simulink model "NonLinearFunction"  (R2021a)
settings: Solver=VariableStepAuto  StartTime=0.0  StopTime=10.0  RelTol=1e-3
settings Model: Creator=Ciro  LastModifiedBy=Ciro

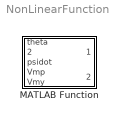
== system NonLinearFunction ==
  MATLAB Function : MATLAB Function  TreatAsAtomicUnit=on

== matlab function NonLinearFunction/MATLAB Function ==
  data: theta input; theta2dot output; thetadot input; psidot input; Vmp input; Vmy input; psi2dot output
function [theta2dot, psi2dot] = fcn(theta,thetadot,psidot,Vmp,Vmy)
theta2dot=(Kpp*Vmp+Kpy*Vmy-Bp*thetadot-Mheli*Lcm^2*sin(theta)*cos(theta)*psidot^2-Mheli*g*Lcm*cos(theta))/Jtp;
psi2dot=(Kyp*Vmp+Kyy*Vmy-By*psidot+2*Mheli*Lcm^2*sin(theta)*cos(theta)*psidot*thetadot)/(Jeq_y+Mheli*Lcm^2*cos(theta)*cos(theta));
end
